simulink model "Discrete_CTC"  (R2020b)
settings: Solver=ode15s  StartTime=0.0  StopTime=119.9  FixedStep=1e-4  RelTol=1e-3  EnableMultiTasking=on
undefined symbols (not defined in the file or in its folder): Kp1, Kp2, Kp3, Kp4, Kp5, Kv1, Kv2, Kv3, Kv4, Kv5, r1, r2, r3, r4, r5, t1, t2, t3, t4, t5
settings Model: Creator=Patricio  LastModifiedBy=patricio
settings DataIOCC: LimitDataPoints=on  SaveFormat=Array  ReturnWorkspaceOutputs=off
settings OptimizationCC: LifeSpan=inf
settings DebuggingCC: UnderspecifiedInitializationDetection=Classic  MergeDetectMultiDrivingBlocksExec=none  SolverPrmCheckMsg=warning  MultiTaskRateTransMsg=warning  StateNameClashWarn=warning  SFUnexpectedBacktrackingDiag=warning  SFNoUnconditionalDefaultTransitionDiag=warning  SFExecutionAtInitializationDiag=none  ArithmeticOperatorsInVariantConditions=warning
settings HardwareCC: ProdBitPerPointer=32  ProdBitPerSizeT=32  ProdBitPerPtrDiffT=32  ProdLargestAtomicFloat=None  ProdIntDivRoundTo=Undefined  ProdEndianess=Unspecified  ProdWordSize=32  ProdHWDeviceType=32-bit Generic
settings ModelReferenceCC: PropagateSignalLabelsOutOfModel=off
settings SFSimCC: SimUseLocalCustomCode=off  CustomCodeUndefinedFunction=UseInterfaceOnly
settings RTWCC: RTWUseLocalCustomCode=off
settings CodeAppCC: StateflowObjectComments=on
settings GRTTargetCC: TargetLangStandard=C89/C90 (ANSI)
settings ConfigComp: CovMetricSettings=dw  CovSaveCumulativeToWorkspaceVar=on  CovSaveSingleToWorkspaceVar=on  CovExternalEMLEnable=off  CovBoundaryAbsTol=1.0e-5

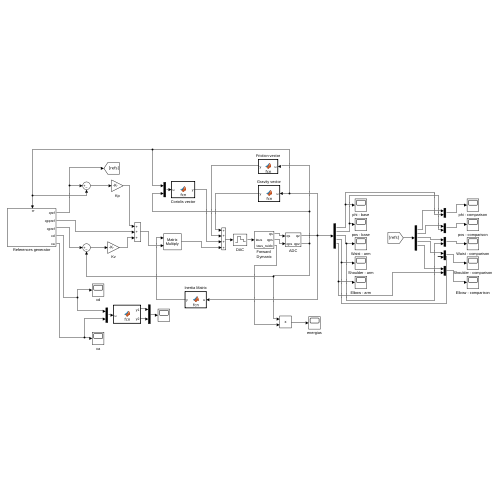
[thumbnail: Simulink's stored preview of the top-level diagram]
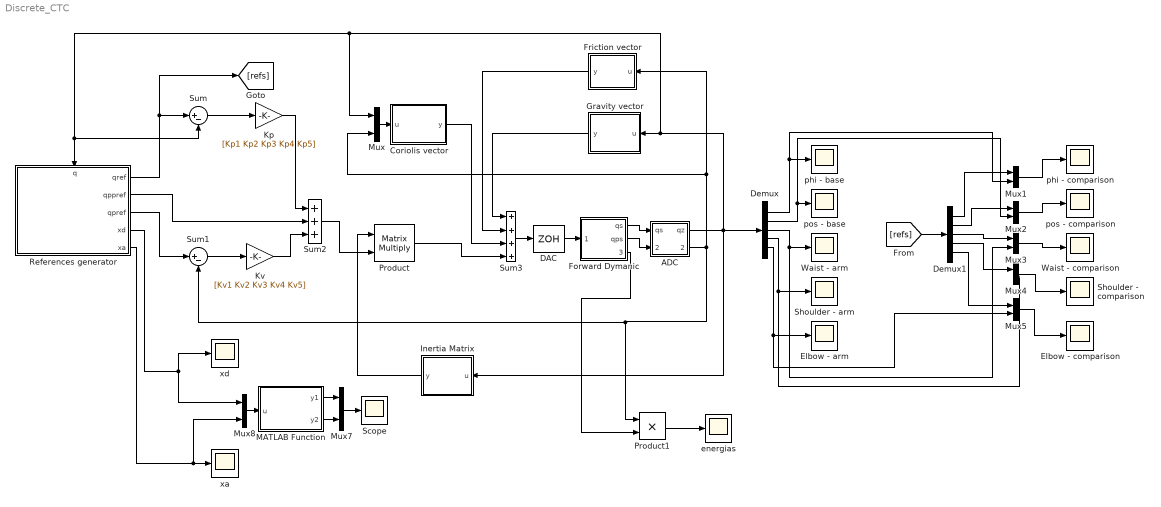
== system Discrete_CTC ==
  ADC : Subsystem
  Coriolis vector : MATLAB Function  TreatAsAtomicUnit=on
  DAC : ZeroOrderHold  SampleTime=1e-3
  Demux : Demux  Outputs=5
  Demux1 : Demux  Outputs=5
  Elbow - arm : Scope
  Elbow - comparison : Scope
  Forward Dymanic : Subsystem
  Friction vector : MATLAB Function  TreatAsAtomicUnit=on
  Gravity vector : MATLAB Function  TreatAsAtomicUnit=on
  Inertia Matrix : MATLAB Function  TreatAsAtomicUnit=on
  Kp : Gain  Gain=[Kp1 Kp2 Kp3 Kp4 Kp5]
  Kv : Gain  Gain=[Kv1 Kv2 Kv3 Kv4 Kv5]
  MATLAB Function : MATLAB Function  TreatAsAtomicUnit=on
  Mux{,1..5,7..8} (8 alike) : Mux  Inputs=2
  Product : Product  Multiplication=Matrix(*)
  Product1 : Product
  References generator : Subsystem
      settings: PortSchema="{\"entries\":[{\"content\":{\"sides\":[{\"content\":{\"connectorIds\":[]},\"type\":\"ConnectorPlacement.EquallySpacedRectSide\",\"uuid\":\"78cd2c92-65ed-4cf8-a1cf-a0f0474b0da8\"},{\"content\":{\"connectorIds\":[\"Out1\",\"Out2\",\"Out3\",\"Out4\",\"Out5\"],\"side\":\"RIGHT\"},\"type\":\"ConnectorPlacement.EquallySpacedRectSide\",\"uuid\":\"ee0b8c83-2e3b-436c-9dc7-32be18272a94\"},{\"content\":{\"connectorIds\":[\"In1\"],\"side\":\"TOP\"},\"type\":\"ConnectorPlacement.EquallySpacedRectSide\",\"uuid\":\"7419595e-10b4-4f6e-bc6b-e1ace5fbe842\"}]},\"type\":\"ConnectorPlacement.EquallySpacedConnector\",\"uuid\":\"acfe5817-2131-4ffc-b257-18a072540c59\"}],\"packageUris\":[\"http://schema.mathworks.com/mf0/Connector/19700101\"],\"version\":\"1.0\"}"
  Scope : Scope
  Shoulder - arm : Scope
  Shoulder - comparison : Scope
  Sum : Sum  Inputs=|+-
  Sum1 : Sum  Inputs=|+-
  Sum2 : Sum  Inputs=+++
  Sum3 : Sum  Inputs=++++
  Waist - arm : Scope
  Waist - comparison : Scope
  energias : Scope
  phi - base : Scope
  phi - comparison : Scope
  pos - base : Scope
  pos - comparison : Scope
  xa : Scope
  xd : Scope
  wires:
  Demux/1 -> Mux1/2, phi - base/1
  Demux/2 -> Mux2/2, pos - base/1
  Demux/3 -> Mux3/2, Waist - arm/1
  Demux/4 -> Mux4/2, Shoulder - arm/1
  Sum/1 -> Kp/1
  Mux/1 -> Coriolis vector/1(u)
  Coriolis vector/1(y) -> Sum3/3
  Product/1 -> Sum3/4
  Gravity vector/1(y) -> Sum3/1
  Sum2/1 -> Product/2
  Inertia Matrix/1(y) -> Product/1
  Sum1/1 -> Kv/1
  Mux1/1 -> phi - comparison/1
  Mux2/1 -> pos - comparison/1
  Mux3/1 -> Waist - comparison/1
  Mux4/1 -> Shoulder - comparison/1
  Mux5/1 -> Elbow - comparison/1
  Demux/5 -> Mux5/2, Elbow - arm/1
  References generator/1(qref) -> [refs], Sum/1
  [refs] -> Demux1/1
  Demux1/1 -> Mux1/1
  Demux1/2 -> Mux2/1
  Demux1/3 -> Mux3/1
  Demux1/4 -> Mux4/1
  Demux1/5 -> Mux5/1
  Kp/1 -> Sum2/1
  Kv/1 -> Sum2/3
  References generator/3(qpref) -> Sum1/1
  References generator/4(xd) -> Mux8/1, xd/1
  References generator/5(xa) -> Mux8/2, xa/1
  References generator/2(qppref) -> Sum2/2
  Product1/1 -> energias/1
  ADC/1(qz) -> Inertia Matrix/1(u), Sum/2, References generator/1(q), Mux/1, Gravity vector/1(u), Demux/1
  Forward Dymanic/1(qs) -> ADC/1(qs)
  Forward Dymanic/2(qps) -> ADC/2(qps)
  ADC/2(qpz) -> Sum1/2, Product1/1, Mux/2, Friction vector/1(u)
  Sum3/1 -> DAC/1
  DAC/1 -> Forward Dymanic/1(taus)
  Forward Dymanic/3(taus_ruido) -> Product1/2
  MATLAB Function/1(y1) -> Mux7/1
  Mux8/1 -> MATLAB Function/1(u)
  MATLAB Function/2(y2) -> Mux7/2
  Mux7/1 -> Scope/1
  Friction vector/1(y) -> Sum3/2

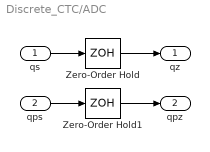
== system Discrete_CTC/ADC ==
  qs : Inport
  qps : Inport  Port=2
  Zero-Order Hold : ZeroOrderHold  SampleTime=1e-3
  Zero-Order Hold1 : ZeroOrderHold  SampleTime=1e-3
  qz : Outport
  qpz : Outport  Port=2
  wires:
  qs/1 -> Zero-Order Hold/1
  Zero-Order Hold/1 -> qz/1
  Zero-Order Hold1/1 -> qpz/1
  qps/1 -> Zero-Order Hold1/1

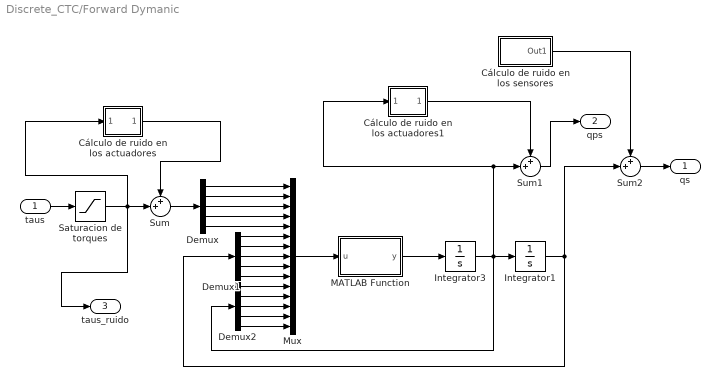
== system Discrete_CTC/Forward Dymanic ==
  taus : Inport
  Cálculo de ruido en los actuadores : Subsystem
  Cálculo de ruido en los actuadores1 : Subsystem
  Cálculo de ruido en los sensores : Subsystem
  Demux : Demux  Outputs=5
  Demux1 : Demux  Outputs=5
  Demux2 : Demux  Outputs=5
  Integrator1 : Integrator  InitialCondition="[0\t0.00100000000000000\t0\t0\t0]"
  Integrator3 : Integrator  InitialCondition=[0 0 0 0 0]  LimitOutput=on  UpperSaturationLimit=[2.4435; 1; 2.2089; 1.19; 1.389]  LowerSaturationLimit=[-2.4435; -1; -2.2089; -1.19; -1.389]
  MATLAB Function : MATLAB Function  TreatAsAtomicUnit=on
  Mux : Mux  Inputs=15
  Saturacion de torques : Saturate  UpperLimit=[10.28; 92.613; 4.732; 4.732; 4.732]  LowerLimit=[-10.28;-92.613;-4.732; -4.732; -4.732]
  Sum : Sum  Inputs=++|
  Sum1 : Sum  Inputs=++|
  Sum2 : Sum  Inputs=++|
  qs : Outport
  qps : Outport  Port=2
  taus_ruido : Outport  Port=3
  wires:
  Demux1/5 -> Mux/10
  Demux1/3 -> Mux/8
  Demux1/1 -> Mux/6
  Demux1/2 -> Mux/7
  Demux1/4 -> Mux/9
  Demux2/1 -> Mux/11
  Demux2/2 -> Mux/12
  Demux2/4 -> Mux/14
  Demux2/5 -> Mux/15
  Demux2/3 -> Mux/13
  Demux/3 -> Mux/3
  Demux/4 -> Mux/4
  Demux/5 -> Mux/5
  Demux/2 -> Mux/2
  Demux/1 -> Mux/1
  Mux/1 -> MATLAB Function/1(u)
  Integrator1/1 -> Sum2/2, Demux1/1
  MATLAB Function/1(y) -> Integrator3/1
  Integrator3/1 -> Cálculo de ruido en los actuadores1/1(vel), Sum1/2, Demux2/1, Integrator1/1
  taus/1 -> Saturacion de torques/1
  Saturacion de torques/1 -> taus_ruido/1, Cálculo de ruido en los actuadores/1(taus), Sum/2
  Sum/1 -> Demux/1
  Sum2/1 -> qs/1
  Sum1/1 -> qps/1
  Cálculo de ruido en los actuadores/1(Out1) -> Sum/1
  Cálculo de ruido en los actuadores1/1(Out1) -> Sum1/1
  Cálculo de ruido en los sensores/1(Out1) -> Sum2/1

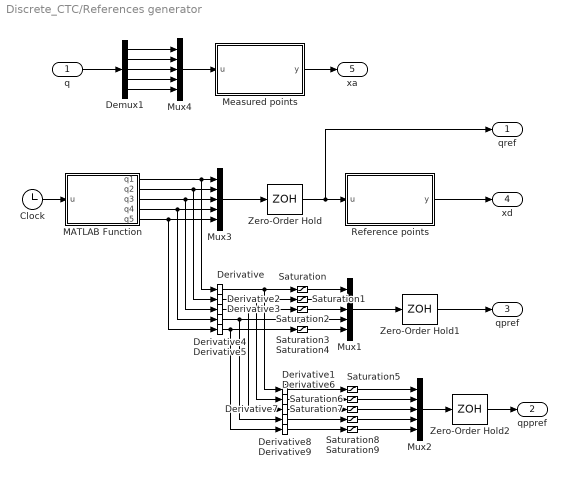
== system Discrete_CTC/References generator ==
  q : Inport
  Clock : Clock
  Demux1 : Demux  Outputs=5
  Derivative{,1..9} (10 alike) : Derivative
  MATLAB Function : MATLAB Function  TreatAsAtomicUnit=on  SystemSampleTime=0.001
  Measured points : MATLAB Function  TreatAsAtomicUnit=on
  Mux{1..4} (4 alike) : Mux  Inputs=5
  Reference points : MATLAB Function  TreatAsAtomicUnit=on
  Saturation : Saturate  UpperLimit=2.4435  LowerLimit=-2.4435
  Saturation1 : Saturate  UpperLimit=1  LowerLimit=-1
  Saturation2 : Saturate  UpperLimit=2.2089  LowerLimit=-2.2089
  Saturation3 : Saturate  UpperLimit=1.19  LowerLimit=-1.19
  Saturation4 : Saturate  UpperLimit=1.389  LowerLimit=-1.389
  Saturation5 : Saturate  UpperLimit=5.236  LowerLimit=-5.236
  Saturation6 : Saturate  UpperLimit=2  LowerLimit=-2
  Saturation7 : Saturate  UpperLimit=12.2718  LowerLimit=-12.2718
  Saturation8 : Saturate  UpperLimit=6.612  LowerLimit=-6.612
  Saturation9 : Saturate  UpperLimit=7.714  LowerLimit=-7.714
  Zero-Order Hold : ZeroOrderHold  SampleTime=1e-3
  Zero-Order Hold1 : ZeroOrderHold  SampleTime=1e-3
  Zero-Order Hold2 : ZeroOrderHold  SampleTime=1e-3
  qref : Outport
  qppref : Outport  Port=2
  qpref : Outport  Port=3
  xd : Outport  Port=4
  xa : Outport  Port=5
  wires:
  Demux1/4 -> Mux4/4
  Demux1/3 -> Mux4/3
  Demux1/1 -> Mux4/1
  Demux1/2 -> Mux4/2
  Demux1/5 -> Mux4/5
  q/1 -> Demux1/1
  Mux4/1 -> Measured points/1(u)
  Measured points/1(y) -> xa/1
  Reference points/1(y) -> xd/1
  Mux3/1 -> Zero-Order Hold/1
  Zero-Order Hold/1 -> qref/1, Reference points/1(u)
  Mux1/1 -> Zero-Order Hold1/1
  Zero-Order Hold1/1 -> qpref/1
  Mux2/1 -> Zero-Order Hold2/1
  Zero-Order Hold2/1 -> qppref/1
  Derivative/1 -> Saturation/1, Derivative1/1
  Saturation3/1 -> Mux1/4
  Derivative4/1 -> Saturation3/1, Derivative8/1
  Derivative2/1 -> Saturation1/1, Derivative6/1
  Saturation/1 -> Mux1/1
  Derivative3/1 -> Saturation2/1, Derivative7/1
  Saturation2/1 -> Mux1/3
  Derivative5/1 -> Saturation4/1, Derivative9/1
  Saturation4/1 -> Mux1/5
  Saturation1/1 -> Mux1/2
  Derivative8/1 -> Saturation8/1
  Derivative9/1 -> Saturation9/1
  Saturation9/1 -> Mux2/5
  Saturation7/1 -> Mux2/3
  Derivative6/1 -> Saturation6/1
  Saturation8/1 -> Mux2/4
  Derivative7/1 -> Saturation7/1
  Derivative1/1 -> Saturation5/1
  Saturation5/1 -> Mux2/1
  Saturation6/1 -> Mux2/2
  MATLAB Function/1(q1) -> Derivative/1, Mux3/1
  MATLAB Function/2(q2) -> Derivative2/1, Mux3/2
  MATLAB Function/3(q3) -> Derivative3/1, Mux3/3
  MATLAB Function/4(q4) -> Derivative4/1, Mux3/4
  MATLAB Function/5(q5) -> Derivative5/1, Mux3/5
  Clock/1 -> MATLAB Function/1(u)

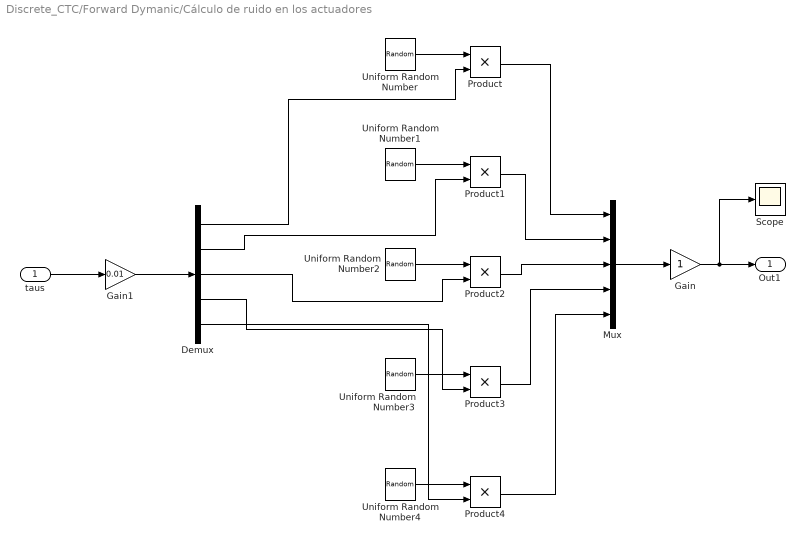
== system Discrete_CTC/Forward Dymanic/Cálculo de ruido en los actuadores ==
  taus : Inport
  Demux : Demux  Outputs=5
  Gain : Gain
  Gain1 : Gain  Gain=0.01
  Mux : Mux  Inputs=5
  Product{,1..4} (5 alike) : Product
  Scope : Scope
  Uniform Random Number : UniformRandomNumber  Seed=t1  SampleTime=0.001
  Uniform Random Number1 : UniformRandomNumber  Seed=t2  SampleTime=0.001
  Uniform Random Number2 : UniformRandomNumber  Seed=t3  SampleTime=0.001
  Uniform Random Number3 : UniformRandomNumber  Seed=t4  SampleTime=0.001
  Uniform Random Number4 : UniformRandomNumber  Seed=t5  SampleTime=0.001
  Out1 : Outport
  wires:
  Demux/5 -> Product4/2
  Demux/4 -> Product3/2
  Demux/3 -> Product2/2
  Demux/2 -> Product1/2
  Demux/1 -> Product/2
  taus/1 -> Gain1/1
  Gain1/1 -> Demux/1
  Uniform Random Number/1 -> Product/1
  Uniform Random Number1/1 -> Product1/1
  Uniform Random Number2/1 -> Product2/1
  Uniform Random Number3/1 -> Product3/1
  Uniform Random Number4/1 -> Product4/1
  Product2/1 -> Mux/3
  Product1/1 -> Mux/2
  Product/1 -> Mux/1
  Product3/1 -> Mux/4
  Product4/1 -> Mux/5
  Mux/1 -> Gain/1
  Gain/1 -> Scope/1, Out1/1

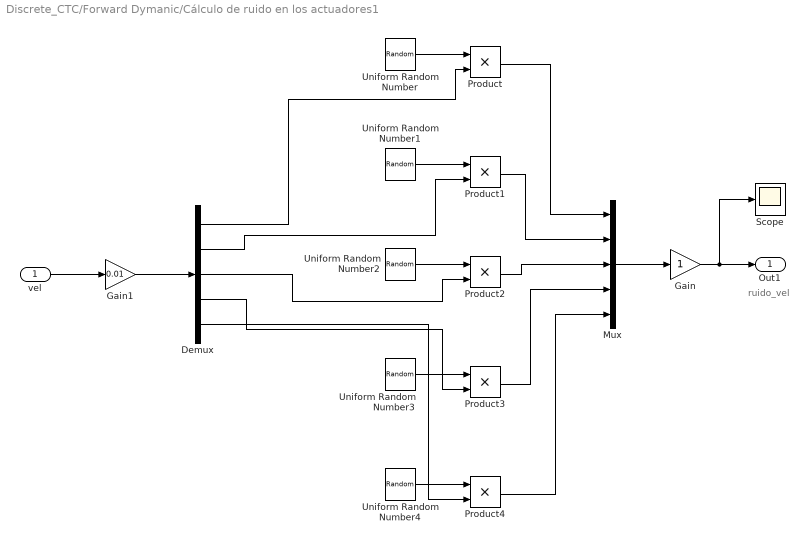
== system Discrete_CTC/Forward Dymanic/Cálculo de ruido en los actuadores1 ==
  note: ruido_vel
  vel : Inport
  Demux : Demux  Outputs=5
  Gain : Gain
  Gain1 : Gain  Gain=0.01
  Mux : Mux  Inputs=5
  Product{,1..4} (5 alike) : Product
  Scope : Scope
  Uniform Random Number : UniformRandomNumber  Seed=t1  SampleTime=0.001
  Uniform Random Number1 : UniformRandomNumber  Seed=t2  SampleTime=0.001
  Uniform Random Number2 : UniformRandomNumber  Seed=t3  SampleTime=0.001
  Uniform Random Number3 : UniformRandomNumber  Seed=t4  SampleTime=0.001
  Uniform Random Number4 : UniformRandomNumber  Seed=t5  SampleTime=0.001
  Out1 : Outport
  wires:
  Gain/1 -> Out1/1, Scope/1
  Mux/1 -> Gain/1
  Product4/1 -> Mux/5
  Product3/1 -> Mux/4
  Product/1 -> Mux/1
  Product1/1 -> Mux/2
  Product2/1 -> Mux/3
  Uniform Random Number4/1 -> Product4/1
  Uniform Random Number3/1 -> Product3/1
  Uniform Random Number2/1 -> Product2/1
  Uniform Random Number1/1 -> Product1/1
  Uniform Random Number/1 -> Product/1
  Gain1/1 -> Demux/1
  vel/1 -> Gain1/1
  Demux/1 -> Product/2
  Demux/2 -> Product1/2
  Demux/3 -> Product2/2
  Demux/4 -> Product3/2
  Demux/5 -> Product4/2

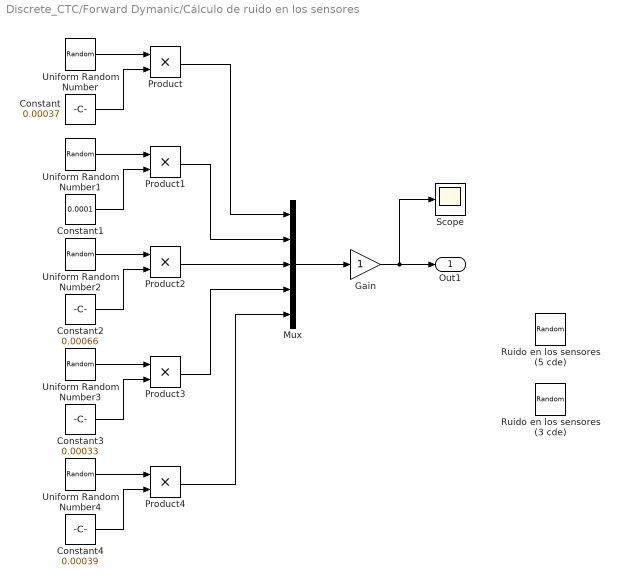
== system Discrete_CTC/Forward Dymanic/Cálculo de ruido en los sensores ==
  Constant : Constant  Value=0.00037
  Constant1 : Constant  Value=0.0001
  Constant2 : Constant  Value=0.00066
  Constant3 : Constant  Value=0.00033
  Constant4 : Constant  Value=0.00039
  Gain : Gain
  Mux : Mux  Inputs=5
  Product{,1..4} (5 alike) : Product
  Ruido en los sensores (3 cde) : UniformRandomNumber  Minimum=[-0.00037 -0.0001 -0.00037 -0.0002 -0.0004]  Maximum=[0.00037 0.0001 0.00037 0.0002 0.0004]  SampleTime=0.1
  Ruido en los sensores (5 cde) : UniformRandomNumber  Minimum=[-0.00037 -0.0001 -0.00066 -0.00033 -0.00039]  Maximum=[0.00037 0.0001 0.00066 0.00033 0.00039]  SampleTime=0.1
  Scope : Scope
  Uniform Random Number : UniformRandomNumber  Seed=r1  SampleTime=0.1
  Uniform Random Number1 : UniformRandomNumber  Seed=r2  SampleTime=0.1
  Uniform Random Number2 : UniformRandomNumber  Seed=r3  SampleTime=0.1
  Uniform Random Number3 : UniformRandomNumber  Seed=r4  SampleTime=0.1
  Uniform Random Number4 : UniformRandomNumber  Seed=r5  SampleTime=0.1
  Out1 : Outport
  wires:
  Constant/1 -> Product/2
  Uniform Random Number/1 -> Product/1
  Uniform Random Number1/1 -> Product1/1
  Constant1/1 -> Product1/2
  Constant2/1 -> Product2/2
  Uniform Random Number2/1 -> Product2/1
  Uniform Random Number3/1 -> Product3/1
  Constant3/1 -> Product3/2
  Constant4/1 -> Product4/2
  Uniform Random Number4/1 -> Product4/1
  Product2/1 -> Mux/3
  Product1/1 -> Mux/2
  Product/1 -> Mux/1
  Product3/1 -> Mux/4
  Product4/1 -> Mux/5
  Mux/1 -> Gain/1
  Gain/1 -> Scope/1, Out1/1

== matlab function Discrete_CTC/Coriolis vector ==
  data: u input size=10; y output size=5
function y = fcn(u)
phi=u(1);
int_vb=u(1);
th3=u(3);
th4=u(4);
th5=u(5);
phip=u(6);
vb=u(7);
th3p=u(8);
th4p=u(9);
th5p=u(10);

%Parámetros de la base
mb=12;		%Masa de la base sin el brazo
Jb=0.5;		%Inercia de la base
b1=1;		%Coeficiente de roce rotacional
b2=0.07;	%Coeficiente de roce lineal

%Parámetros del brazo
m3=2.867;
m4=0.633;
m5=0.79;
r3=0.025;	%pag 39 pdf Katana
L3=0.06;
L4=0.19;
L5=0.139;
b3=0.12;
b4=0.12;
b5=0.12;
g=9.8062;
 
C1 =(L5^2*m5*th3p*th4p*sin(th4))/3 - (L5^2*m5*th3p*th4p*cos(th5)^2*sin(th4))/3 + L4*m4*phip*vb*cos(th3)*cos(th4) + 2*L4*m5*phip*vb*cos(th3)*cos(th4) - (L4*L5*m5*th3p*th4p*cos(th4)*sin(th5))/2 + L5*m5*phip*vb*cos(th3)*cos(th4)*cos(th5) - L5*m5*phip*vb*cos(th3)*sin(th4)*sin(th5) - (L5^2*m5*th3p*th4p*cos(th4)*cos(th5)*sin(th5))/3;
C2 =(L5*m5*th5p^2*cos(th3)*sin(th4)*sin(th5))/2 - L4*m5*th4p^2*cos(th3)*cos(th4) - (L5*m5*th5p^2*cos(th3)*cos(th4)*cos(th5))/2 - (L4*m4*th4p^2*cos(th3)*cos(th4))/2 + (L5*m5*th3p*th4p*sin(th3)*sin(th5))/2;
C3 =(L5^2*m5*th3p*th4p*sin(th4))/3 - (L5^2*m5*th3p*th4p*cos(th5)^2*sin(th4))/3 + L4*m4*phip*vb*cos(th3)*cos(th4) + 2*L4*m5*phip*vb*cos(th3)*cos(th4) - (L4*L5*m5*th3p*th4p*cos(th4)*sin(th5))/2 + L5*m5*phip*vb*cos(th3)*cos(th4)*cos(th5) - L5*m5*phip*vb*cos(th3)*sin(th4)*sin(th5) - (L5^2*m5*th3p*th4p*cos(th4)*cos(th5)*sin(th5))/3;
C4 =(L4*L5*m5*sin(th5)*th4p^2)/2 - (L4*L5*m5*th5p^2*sin(th5))/2 - L4*m4*phip*vb*sin(th3)*sin(th4) - 2*L4*m5*phip*vb*sin(th3)*sin(th4) - L5*m5*phip*vb*cos(th4)*sin(th3)*sin(th5) - L5*m5*phip*vb*cos(th5)*sin(th3)*sin(th4);
C5 =-(L5*m5*(- L4*sin(th5)*th4p^2 + 2*phip*vb*cos(th4)*sin(th3)*sin(th5) + 2*phip*vb*cos(th5)*sin(th3)*sin(th4)))/2;
 
C=[C1;C2;C3;C4;C5];
y=C;

== matlab function Discrete_CTC/Forward Dymanic/MATLAB Function ==
  data: u input size=15; y output size=5
function y = fcn(u)
tau1=u(1);
flin1=u(2);
tau3=u(3);
tau4=u(4);
tau5=u(5);
phi=u(6);
int_vb=u(7);
th3=u(8);
th4=u(9);
th5=u(10);
phip=u(11);
vb=u(12);
th3p=u(13);
th4p=u(14);
th5p=u(15);

%Parameters:

%Mobile base
mb=12;		%Mass without arm
Jb=0.5;		%Izz in base frame
b1=1;		%Rotational friction coefficient measured in the laboratory
b2=0.07;	%Lineal friction coefficient measured in the laboratory

%Arm
m3=2.867;
m4=0.633;
m5=0.79;
r3=0.025;	%Katana page 39 of manual
L3=0.06;
L4=0.19;
L5=0.139;
b3=0.12;
b4=0.12;
b5=0.12;
g=9.8062;

M11 =Jb + (L3^2*m3)/12 + (L4^2*m4)/6 + (L4^2*m5)/2 + (L5^2*m5)/6 + (L4^2*m4*cos(2*th4))/6 + (L4^2*m5*cos(2*th4))/2 + (L5^2*m5*cos(2*th4 + 2*th5))/6 + (L4*L5*m5*cos(th5))/2 + (L4*L5*m5*cos(2*th4 + th5))/2;
M12 =-(sin(th3)*(L5*m5*cos(th4 + th5) + L4*m4*cos(th4) + 2*L4*m5*cos(th4)))/2;
M13 =(L3^2*m3)/12 + (L4^2*m4)/6 + (L4^2*m5)/2 + (L5^2*m5)/6 + (L4^2*m4*cos(2*th4))/6 + (L4^2*m5*cos(2*th4))/2 + (L5^2*m5*cos(2*th4 + 2*th5))/6 + (L4*L5*m5*cos(th5))/2 + (L4*L5*m5*cos(2*th4 + th5))/2;
M14 =0;
M15 =0;

M21 =-(sin(th3)*(L5*m5*cos(th4 + th5) + L4*m4*cos(th4) + 2*L4*m5*cos(th4)))/2;
M22 =m3 + m4 + m5 + 2*mb;
M23 =-(sin(th3)*(L5*m5*cos(th4 + th5) + L4*m4*cos(th4) + 2*L4*m5*cos(th4)))/2;
M24 =-(cos(th3)*(L4*m4*sin(th4) + 2*L4*m5*sin(th4) + L5*m5*sin(th4 + th5)))/2;
M25 =-(L5*m5*sin(th4 + th5)*cos(th3))/2;
 
M31 =(L3^2*m3)/12 + (L4^2*m4)/6 + (L4^2*m5)/2 + (L5^2*m5)/6 + (L4^2*m4*cos(2*th4))/6 + (L4^2*m5*cos(2*th4))/2 + (L5^2*m5*cos(2*th4 + 2*th5))/6 + (L4*L5*m5*cos(th5))/2 + (L4*L5*m5*cos(2*th4 + th5))/2;
M32 =-(sin(th3)*(L5*m5*cos(th4 + th5) + L4*m4*cos(th4) + 2*L4*m5*cos(th4)))/2;
M33 =(L3^2*m3)/12 + (L4^2*m4)/6 + (L4^2*m5)/2 + (L5^2*m5)/6 + (L4^2*m4*cos(2*th4))/6 + (L4^2*m5*cos(2*th4))/2 + (L5^2*m5*cos(2*th4 + 2*th5))/6 + (L4*L5*m5*cos(th5))/2 + (L4*L5*m5*cos(2*th4 + th5))/2;
M34 =0;
M35 =0;

M41 =0;
M42 =-(cos(th3)*(L4*m4*sin(th4) + 2*L4*m5*sin(th4) + L5*m5*sin(th4 + th5)))/2;
M43 =0;
M44 =(L4^2*m4)/3 + L4^2*m5 + (L5^2*m5)/3 + L4*L5*m5*cos(th5);
M45 =(L5*m5*(2*L5 + 3*L4*cos(th5)))/6;

M51 =0;
M52 =-(L5*m5*sin(th4 + th5)*cos(th3))/2;
M53 =0;
M54 =(L5*m5*(2*L5 + 3*L4*cos(th5)))/6;
M55 =(L5^2*m5)/3;
 
C1 =(L4*m4*phip*vb*cos(th3 - th4))/2 + L4*m5*phip*vb*cos(th3 - th4) + (L5*m5*phip*vb*cos(th3 + th4 + th5))/2 + (L5^2*m5*phip*th4p*sin(th4))/6 + (L5^2*m5*phip*th5p*sin(th5))/6 + (L5^2*m5*th3p*th4p*sin(th4))/6 + (L5^2*m5*th3p*th5p*sin(th5))/6 - (L5^2*m5*phip*th4p*sin(th4 + 2*th5))/6 - (L5^2*m5*phip*th5p*sin(2*th4 + th5))/6 - (L5^2*m5*th3p*th4p*sin(th4 + 2*th5))/6 - (L5^2*m5*th3p*th5p*sin(2*th4 + th5))/6 - (L4^2*m4*phip*th4p*sin(2*th4))/6 - (L4^2*m5*phip*th4p*sin(2*th4))/2 - (L4^2*m4*th3p*th4p*sin(2*th4))/6 - (L4^2*m5*th3p*th4p*sin(2*th4))/2 + (L4*m4*phip*vb*cos(th3 + th4))/2 + L4*m5*phip*vb*cos(th3 + th4) - (L5^2*m5*phip*th4p*sin(2*th4 + 2*th5))/6 - (L5^2*m5*phip*th5p*sin(2*th4 + 2*th5))/6 - (L5^2*m5*th3p*th4p*sin(2*th4 + 2*th5))/6 - (L5^2*m5*th3p*th5p*sin(2*th4 + 2*th5))/6 + (L5*m5*phip*vb*cos(th3 - th4 - th5))/2 - (L4*L5*m5*phip*th4p*sin(th4 + th5))/4 - (L4*L5*m5*th3p*th4p*sin(th4 + th5))/4 - (L4*L5*m5*phip*th5p*sin(th5))/4 - (L4*L5*m5*th3p*th5p*sin(th5))/4 + (L4*L5*m5*phip*th4p*sin(th4 - th5))/4 - (L4*L5*m5*phip*th4p*sin(2*th4 + th5))/2 - (L4*L5*m5*phip*th5p*sin(2*th4 + th5))/4 + (L4*L5*m5*th3p*th4p*sin(th4 - th5))/4 - (L4*L5*m5*th3p*th4p*sin(2*th4 + th5))/2 - (L4*L5*m5*th3p*th5p*sin(2*th4 + th5))/4 - (L4*L5*m5*phip*th5p*sin(2*th4))/4 - (L4*L5*m5*th3p*th5p*sin(2*th4))/4;
C2 =(L5*m5*phip^2*cos(th3)*sin(th4)*sin(th5))/2 - L4*m5*phip^2*cos(th3)*cos(th4) - (L4*m4*th3p^2*cos(th3)*cos(th4))/2 - (L4*m4*th4p^2*cos(th3)*cos(th4))/2 - L4*m5*th3p^2*cos(th3)*cos(th4) - L4*m5*th4p^2*cos(th3)*cos(th4) - (L5*m5*phip^2*cos(th3)*cos(th4)*cos(th5))/2 - (L5*m5*th3p^2*cos(th3)*cos(th4)*cos(th5))/2 - (L5*m5*th4p^2*cos(th3)*cos(th4)*cos(th5))/2 - (L5*m5*th5p^2*cos(th3)*cos(th4)*cos(th5))/2 - (L4*m4*phip^2*cos(th3)*cos(th4))/2 + (L5*m5*th3p^2*cos(th3)*sin(th4)*sin(th5))/2 + (L5*m5*th4p^2*cos(th3)*sin(th4)*sin(th5))/2 + (L5*m5*th5p^2*cos(th3)*sin(th4)*sin(th5))/2 - L4*m4*phip*th3p*cos(th3)*cos(th4) - 2*L4*m5*phip*th3p*cos(th3)*cos(th4) + (L4*m4*phip*th4p*sin(th3)*sin(th4))/2 + L4*m5*phip*th4p*sin(th3)*sin(th4) + (L5*m5*phip*th4p*sin(th3)*sin(th5))/2 + (L5*m5*phip*th5p*sin(th3)*sin(th4))/2 + (L4*m4*th3p*th4p*sin(th3)*sin(th4))/2 + L4*m5*th3p*th4p*sin(th3)*sin(th4) + (L5*m5*th3p*th4p*sin(th3)*sin(th5))/2 + (L5*m5*th3p*th5p*sin(th3)*sin(th4))/2 - L5*m5*phip*th3p*cos(th3)*cos(th4)*cos(th5) - L5*m5*th4p*th5p*cos(th3)*cos(th4)*cos(th5) + L5*m5*phip*th3p*cos(th3)*sin(th4)*sin(th5) + (L5*m5*phip*th4p*cos(th4)*sin(th3)*sin(th5))/2 + (L5*m5*phip*th4p*cos(th5)*sin(th3)*sin(th4))/2 + (L5*m5*phip*th5p*cos(th4)*sin(th3)*sin(th5))/2 + (L5*m5*phip*th5p*cos(th5)*sin(th3)*sin(th4))/2 + (L5*m5*th3p*th4p*cos(th4)*sin(th3)*sin(th5))/2 + (L5*m5*th3p*th4p*cos(th5)*sin(th3)*sin(th4))/2 + (L5*m5*th3p*th5p*cos(th4)*sin(th3)*sin(th5))/2 + (L5*m5*th3p*th5p*cos(th5)*sin(th3)*sin(th4))/2 + L5*m5*th4p*th5p*cos(th3)*sin(th4)*sin(th5);
C3 =(L4*m4*phip*vb*cos(th3 - th4))/2 + L4*m5*phip*vb*cos(th3 - th4) + (L5*m5*phip*vb*cos(th3 + th4 + th5))/2 + (L5^2*m5*phip*th4p*sin(th4))/6 + (L5^2*m5*phip*th5p*sin(th5))/6 + (L5^2*m5*th3p*th4p*sin(th4))/6 + (L5^2*m5*th3p*th5p*sin(th5))/6 - (L5^2*m5*phip*th4p*sin(th4 + 2*th5))/6 - (L5^2*m5*phip*th5p*sin(2*th4 + th5))/6 - (L5^2*m5*th3p*th4p*sin(th4 + 2*th5))/6 - (L5^2*m5*th3p*th5p*sin(2*th4 + th5))/6 - (L4^2*m4*phip*th4p*sin(2*th4))/6 - (L4^2*m5*phip*th4p*sin(2*th4))/2 - (L4^2*m4*th3p*th4p*sin(2*th4))/6 - (L4^2*m5*th3p*th4p*sin(2*th4))/2 + (L4*m4*phip*vb*cos(th3 + th4))/2 + L4*m5*phip*vb*cos(th3 + th4) - (L5^2*m5*phip*th4p*sin(2*th4 + 2*th5))/6 - (L5^2*m5*phip*th5p*sin(2*th4 + 2*th5))/6 - (L5^2*m5*th3p*th4p*sin(2*th4 + 2*th5))/6 - (L5^2*m5*th3p*th5p*sin(2*th4 + 2*th5))/6 + (L5*m5*phip*vb*cos(th3 - th4 - th5))/2 - (L4*L5*m5*phip*th4p*sin(th4 + th5))/4 - (L4*L5*m5*th3p*th4p*sin(th4 + th5))/4 - (L4*L5*m5*phip*th5p*sin(th5))/4 - (L4*L5*m5*th3p*th5p*sin(th5))/4 + (L4*L5*m5*phip*th4p*sin(th4 - th5))/4 - (L4*L5*m5*phip*th4p*sin(2*th4 + th5))/2 - (L4*L5*m5*phip*th5p*sin(2*th4 + th5))/4 + (L4*L5*m5*th3p*th4p*sin(th4 - th5))/4 - (L4*L5*m5*th3p*th4p*sin(2*th4 + th5))/2 - (L4*L5*m5*th3p*th5p*sin(2*th4 + th5))/4 - (L4*L5*m5*phip*th5p*sin(2*th4))/4 - (L4*L5*m5*th3p*th5p*sin(2*th4))/4;
C4 =(L4^2*m4*phip^2*sin(2*th4))/6 + (L4^2*m5*phip^2*sin(2*th4))/2 + (L4^2*m4*th3p^2*sin(2*th4))/6 + (L4^2*m5*th3p^2*sin(2*th4))/2 + (L5^2*m5*phip^2*sin(2*th4 + 2*th5))/6 + (L5^2*m5*th3p^2*sin(2*th4 + 2*th5))/6 - (L4*m4*phip*vb*cos(th3 - th4))/2 - L4*m5*phip*vb*cos(th3 - th4) + (L5*m5*phip*vb*cos(th3 + th4 + th5))/2 - (L4*L5*m5*th5p^2*sin(th5))/2 + (L4*L5*m5*phip^2*sin(2*th4 + th5))/2 + (L4*L5*m5*th3p^2*sin(2*th4 + th5))/2 + (L4^2*m4*phip*th3p*sin(2*th4))/3 + L4^2*m5*phip*th3p*sin(2*th4) + (L4*m4*phip*vb*cos(th3 + th4))/2 + L4*m5*phip*vb*cos(th3 + th4) + (L5^2*m5*phip*th3p*sin(2*th4 + 2*th5))/3 - (L5*m5*phip*vb*cos(th3 - th4 - th5))/2 - L4*L5*m5*th4p*th5p*sin(th5) + L4*L5*m5*phip*th3p*sin(2*th4 + th5);
C5 =(L5*m5*(3*L4*phip^2*sin(th5) - 6*phip*vb*cos(th3 - th4 - th5) + 6*phip*vb*cos(th3 + th4 + th5) + 3*L4*th3p^2*sin(th5) + 6*L4*th4p^2*sin(th5) + 3*L4*phip^2*sin(2*th4 + th5) + 3*L4*th3p^2*sin(2*th4 + th5) + 2*L5*phip^2*sin(2*th4 + 2*th5) + 2*L5*th3p^2*sin(2*th4 + 2*th5) + 4*L5*phip*th3p*sin(2*th4 + 2*th5) + 6*L4*phip*th3p*sin(th5) + 6*L4*phip*th3p*sin(2*th4 + th5)))/12;
 
G1=0;
G2=0;
G3=0;
G4= (L5*m5*cos(th4 + th5))/2 + (L4*m4*cos(th4))/2 + L4*m5*cos(th4);
G5= (L5*m5*cos(th4 + th5))/2;

F1=b1*phip;
F2=b2*vb;
F3=b3*th3p;
F4=b4*th4p;
F5=b5*th5p;
M=[M11 M12 M13 M14 M15;
   M21 M22 M23 M24 M25;
   M31 M32 M33 M34 M35;
   M41 M42 M43 M44 M45;
   M51 M52 M53 M54 M55];
C=[C1;C2;C3;C4;C5];
G=[G1;G2;G3;G4;G5];
F=[F1;F2;F3;F4;F5];
tau=[tau1;flin1;tau3;tau4;tau5];
qpp=M\(tau-C-F-G*g);
y=qpp;

== matlab function Discrete_CTC/Friction vector ==
  data: u input size=5; y output size=5
function y = fcn(u)
phip=u(1);
vb=u(2);
th3p=u(3);
th4p=u(4);
th5p=u(5);

%Parámetros:

%Parámetros de la base
b1=1;		%Coeficiente de roce rotacional
b2=0.07;	%Coeficiente de roce lineal

%Parámetros del brazo
b3=0.12;
b4=0.12;
b5=0.12;

F1=b1*phip;
F2=b2*vb;
F3=b3*th3p;
F4=b4*th4p;
F5=b5*th5p;
F=[F1;F2;F3;F4;F5];
y=F;

== matlab function Discrete_CTC/Inertia Matrix ==
  data: u input size=5; y output size=[5,5]
function y = fcn(u)
phi=u(1);
int_vb=u(2);
th3=u(3);
th4=u(4);
th5=u(5);

%Parámetros de la base
mb=12;		%Masa de la base sin el brazo
Jb=0.5;		%Inercia de la base
b1=1;		%Coeficiente de roce rotacional
b2=0.07;	%Coeficiente de roce lineal

%Parámetros del brazo
m3=2.867;
m4=0.633;
m5=0.79;
r3=0.025;	%pag 39 pdf Katana
L3=0.06;
L4=0.19;
L5=0.139;
b3=0.12;
b4=0.12;
b5=0.12;
g=9.8062;

M11 =Jb + (L3^2*m3)/12 + (L4^2*m4)/6 + (L4^2*m5)/2 + (L5^2*m5)/6 + (L4^2*m4*cos(2*th4))/6 + (L4^2*m5*cos(2*th4))/2 + (L5^2*m5*cos(2*th4 + 2*th5))/6 + (L4*L5*m5*cos(th5))/2 + (L4*L5*m5*cos(2*th4 + th5))/2;
M12 =-(sin(th3)*(L5*m5*cos(th4 + th5) + L4*m4*cos(th4) + 2*L4*m5*cos(th4)))/2;
M13 =(L3^2*m3)/12 + (L4^2*m4)/6 + (L4^2*m5)/2 + (L5^2*m5)/6 + (L4^2*m4*cos(2*th4))/6 + (L4^2*m5*cos(2*th4))/2 + (L5^2*m5*cos(2*th4 + 2*th5))/6 + (L4*L5*m5*cos(th5))/2 + (L4*L5*m5*cos(2*th4 + th5))/2;
M14 =0;
M15 =0;

M21 =-(sin(th3)*(L5*m5*cos(th4 + th5) + L4*m4*cos(th4) + 2*L4*m5*cos(th4)))/2;
M22 =m3 + m4 + m5 + 2*mb;
M23 =-(sin(th3)*(L5*m5*cos(th4 + th5) + L4*m4*cos(th4) + 2*L4*m5*cos(th4)))/2;
M24 =-(cos(th3)*(L4*m4*sin(th4) + 2*L4*m5*sin(th4) + L5*m5*sin(th4 + th5)))/2;
M25 =-(L5*m5*sin(th4 + th5)*cos(th3))/2;
 
M31 =(L3^2*m3)/12 + (L4^2*m4)/6 + (L4^2*m5)/2 + (L5^2*m5)/6 + (L4^2*m4*cos(2*th4))/6 + (L4^2*m5*cos(2*th4))/2 + (L5^2*m5*cos(2*th4 + 2*th5))/6 + (L4*L5*m5*cos(th5))/2 + (L4*L5*m5*cos(2*th4 + th5))/2;
M32 =-(sin(th3)*(L5*m5*cos(th4 + th5) + L4*m4*cos(th4) + 2*L4*m5*cos(th4)))/2;
M33 =(L3^2*m3)/12 + (L4^2*m4)/6 + (L4^2*m5)/2 + (L5^2*m5)/6 + (L4^2*m4*cos(2*th4))/6 + (L4^2*m5*cos(2*th4))/2 + (L5^2*m5*cos(2*th4 + 2*th5))/6 + (L4*L5*m5*cos(th5))/2 + (L4*L5*m5*cos(2*th4 + th5))/2;
M34 =0;
M35 =0;

M41 =0;
M42 =-(cos(th3)*(L4*m4*sin(th4) + 2*L4*m5*sin(th4) + L5*m5*sin(th4 + th5)))/2;
M43 =0;
M44 =(L4^2*m4)/3 + L4^2*m5 + (L5^2*m5)/3 + L4*L5*m5*cos(th5);
M45 =(L5*m5*(2*L5 + 3*L4*cos(th5)))/6;

M51 =0;
M52 =-(L5*m5*sin(th4 + th5)*cos(th3))/2;
M53 =0;
M54 =(L5*m5*(2*L5 + 3*L4*cos(th5)))/6;
M55 =(L5^2*m5)/3;
 
M=[M11 M12 M13 M14 M15;
   M21 M22 M23 M24 M25;
   M31 M32 M33 M34 M35;
   M41 M42 M43 M44 M45;
   M51 M52 M53 M54 M55];

y=M;

== matlab function Discrete_CTC/Gravity vector ==
  data: u input size=5; y output size=5
function y = fcn(u)
% Entradas
phi=u(1);
int_vb=u(2);
th3=u(3);
th4=u(4);
th5=u(5);

%Parámetros de la base
mb=12;		%Masa de la base sin el brazo
Jb=0.5;		%Inercia de la base
b1=1;		%Coeficiente de roce rotacional
b2=0.07;	%Coeficiente de roce lineal

%Parámetros del brazo
m3=2.867;
m4=0.633;
m5=0.79;
r3=0.025;	%pag 39 pdf Katana
L3=0.06;
L4=0.19;
L5=0.139;
b3=0.12;
b4=0.12;
b5=0.12;
g=9.8062;

G1=0;
G2=0;
G3=0;
G4= (L5*m5*cos(th4 + th5))/2 + (L4*m4*cos(th4))/2 + L4*m5*cos(th4);
G5= (L5*m5*cos(th4 + th5))/2;

G=[G1;G2;G3;G4;G5];
y=G*g;

== matlab function Discrete_CTC/References generator/MATLAB Function ==
  data: u input; q1 output; q2 output; q3 output; q4 output; q5 output
function [q1,q2,q3,q4,q5] = fcn(u)
%#codegen
% Trajectory interpolation function for Simulink.
% The trajectory MAT-file used in the load() call below will be
% programmatically updated by run_trajectory_experiments.m before
% each experiment.

persistent i q
t = u;

if isempty(i)
    i = 1;
end

if isempty(q)
    % This line will be edited by the main script:
    q = load('PLACEHOLDER_TRAJ.mat');
end

ts = 0.1;
if (t > 0) && (mod(t, ts) == 0)
    i = i + 1;
end

% Bound index to available rows
n_rows = size(q.q, 1);
if i > n_rows
    i = n_rows;
end

q1 = q.q(i, 1);
q2 = q.q(i, 2);
q3 = q.q(i, 3);
q4 = q.q(i, 4);
q5 = q.q(i, 5);
end

== matlab function Discrete_CTC/References generator/Reference points ==
  data: u input; y output
function y = fcn(u)
q1=u(1);
q2=u(2);
q3=u(3);
q4=u(4);
q5=u(5);
y=cal_cindir(q1,q2,q3,q4,q5);

== matlab function Discrete_CTC/References generator/Measured points ==
  data: u input; y output
function y = fcn(u)
q1=u(1);
q2=u(2);
q3=u(3);
q4=u(4);
q5=u(5);
y=cal_cindir(q1,q2,q3,q4,q5);

== matlab function Discrete_CTC/MATLAB Function ==
  data: u input size=6; y1 output; y2 output
function [y1,y2] = fcn(u)
xref=[u(1);u(2);u(3)];
xmed=[u(4);u(5);u(6)];
y1=norm(xref);
y2=norm(xmed);
